simulink model "cartpole"  (R2021a)
settings: Solver=FixedStepAuto  StartTime=0.0  StopTime=T_end  FixedStep=Tsim  RelTol=1e-3
values from neighbouring files (symbols this model uses):
  r1 = const(1)    [loop_loader.m]
  r2 = const(2)    [loop_loader.m]
  Ts = 1e-2    (= 0.01)    [loop_loader.m]
undefined symbols (not defined in the file or in its folder): A, B, C, K_lqr, P_k_init, q1, q2, Q_ctrl, R_ctrl, x0
libraries: simulink x4
settings Model: Creator=rodpod21  LastModifiedBy=rodpod21

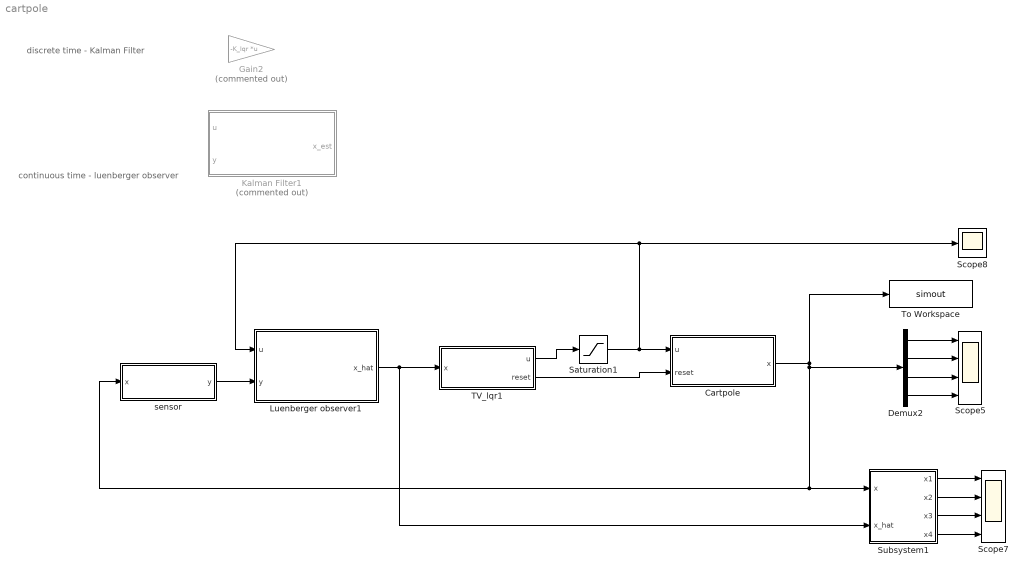
== system cartpole ==
  note: continuous time - luenberger observer
  note: discrete time - Kalman Filter
  Cartpole : Subsystem
  Demux2 : Demux
  Gain2 : Gain  Commented=on  Gain=-K_lqr  Multiplication=Matrix(K*u)
  Kalman Filter1 : Subsystem  Commented=on  TreatAsAtomicUnit=on  SystemSampleTime=Ts
  Luenberger observer1 : Subsystem
  Saturation1 : Saturate  UpperLimit=10  LowerLimit=-10
  Scope5 : Scope  NumInputPorts=4
  Scope7 : Scope  NumInputPorts=4
  Scope8 : Scope
  Subsystem1 : Subsystem
  TV_lqr1 : Subsystem  TreatAsAtomicUnit=on  SystemSampleTime=Ts
  To Workspace : ToWorkspace  VariableName=simout  SaveFormat=Timeseries  SampleTime=-1
  sensor : Subsystem
  wires:
  Subsystem1/1(x1) -> Scope7/1
  Subsystem1/3(x3) -> Scope7/3
  Subsystem1/4(x4) -> Scope7/4
  Subsystem1/2(x2) -> Scope7/2
  Demux2/4 -> Scope5/4
  Demux2/3 -> Scope5/3
  Demux2/2 -> Scope5/2
  Demux2/1 -> Scope5/1
  Saturation1/1 -> Cartpole/1(u), Scope8/1, Luenberger observer1/1(u)
  Luenberger observer1/1(x_hat) -> TV_lqr1/1(x), Subsystem1/2(x_hat)
  sensor/1(y) -> Luenberger observer1/2(y)
  TV_lqr1/1(u) -> Saturation1/1
  Cartpole/1(x) -> To Workspace/1, sensor/1(x), Subsystem1/1(x), Demux2/1
  TV_lqr1/2(reset) -> Cartpole/2(reset)

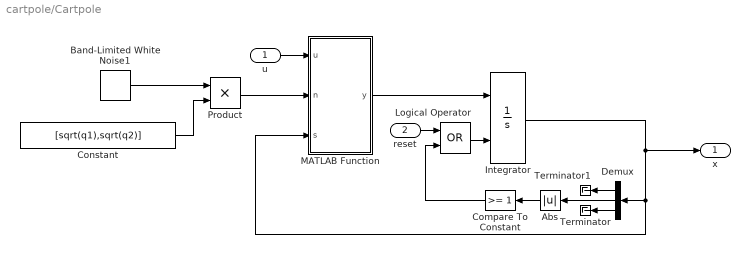
== system cartpole/Cartpole ==
  u : Inport
  reset : Inport  Port=2
  Abs : Abs
  Band-Limited White Noise1 : simulink/Sources/Band-Limited White Noise  Cov=[1,1]  Ts=Ts  seed=[23341]
  Compare To Constant : simulink/Logic and Bit Operations/Compare To Constant  relop=>=  const=1  OutDataTypeStr=boolean
  Constant : Constant  Value=[sqrt(q1),sqrt(q2)]
  Demux : Demux  Outputs=[2,1,1]
  Integrator : Integrator  ExternalReset=rising  InitialCondition=x0
  Logical Operator : Logic  Operator=OR  AllPortsSameDT=off  OutDataTypeStr=boolean
  MATLAB Function : MATLAB Function  TreatAsAtomicUnit=on
  Product : Product
  Terminator : Terminator
  Terminator1 : Terminator
  x : Outport
  wires:
  MATLAB Function/1(y) -> Integrator/1
  Integrator/1 -> x/1, MATLAB Function/3(s), Demux/1
  u/1 -> MATLAB Function/1(u)
  Band-Limited White Noise1/1 -> Product/1
  Product/1 -> MATLAB Function/2(n)
  Compare To Constant/1 -> Logical Operator/2
  Demux/3 -> Terminator/1
  Demux/1 -> Terminator1/1
  Demux/2 -> Abs/1
  Abs/1 -> Compare To Constant/1
  Logical Operator/1 -> Integrator/2
  reset/1 -> Logical Operator/1
  Constant/1 -> Product/2

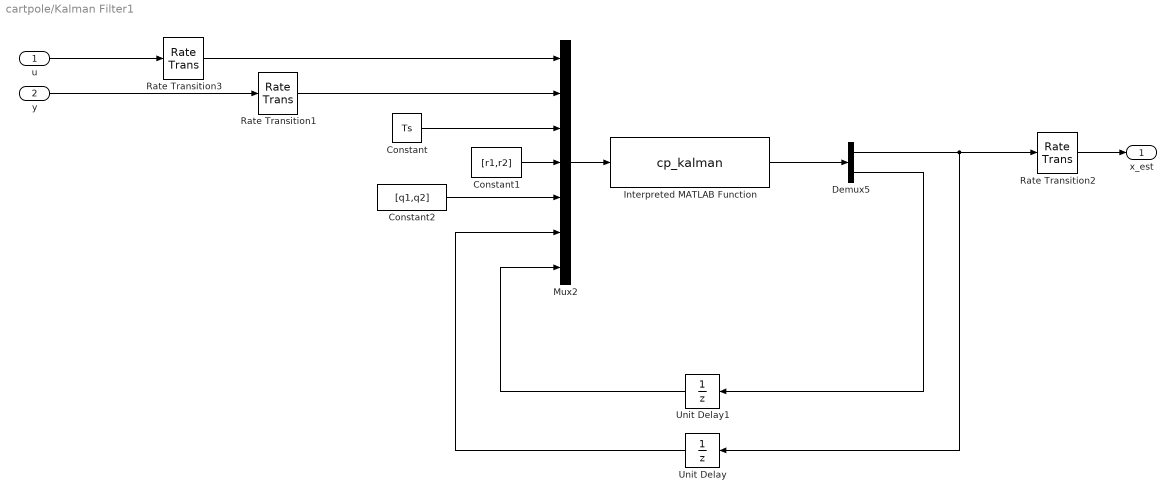
== system cartpole/Kalman Filter1 ==
  u : Inport
  y : Inport  Port=2
  Constant : Constant  Value=Ts
  Constant1 : Constant  Value=[r1,r2]
  Constant2 : Constant  Value=[q1,q2]
  Demux5 : Demux  Outputs=[4, 16]
  Interpreted MATLAB Function : MATLABFcn  MATLABFcn=cp_kalman  OutputDimensions=20
  Mux2 : Mux  Inputs=7
  Rate Transition1 : RateTransition  OutPortSampleTime=Ts
  Rate Transition2 : RateTransition
  Rate Transition3 : RateTransition  OutPortSampleTime=Ts
  Unit Delay : UnitDelay  InitialCondition=x0  SampleTime=-1  HasFrameUpgradeWarning=on
  Unit Delay1 : UnitDelay  InitialCondition=reshape( P_k_init*eye(4),[16,1])  SampleTime=-1  HasFrameUpgradeWarning=on
  x_est : Outport
  wires:
  Unit Delay1/1 -> Mux2/7
  Demux5/1 -> Rate Transition2/1, Unit Delay/1
  y/1 -> Rate Transition1/1
  Demux5/2 -> Unit Delay1/1
  Interpreted MATLAB Function/1 -> Demux5/1
  u/1 -> Rate Transition3/1
  Unit Delay/1 -> Mux2/6
  Mux2/1 -> Interpreted MATLAB Function/1
  Constant/1 -> Mux2/3
  Constant1/1 -> Mux2/4
  Constant2/1 -> Mux2/5
  Rate Transition3/1 -> Mux2/1
  Rate Transition1/1 -> Mux2/2
  Rate Transition2/1 -> x_est/1

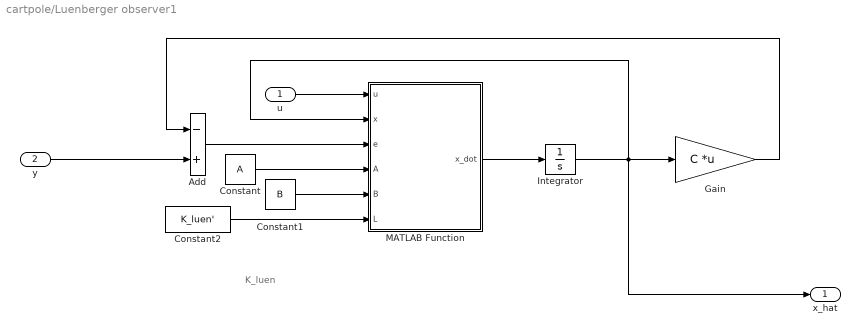
== system cartpole/Luenberger observer1 ==
  note: K_luen
  u : Inport
  y : Inport  Port=2
  Add : Sum  Inputs=-+
  Constant : Constant  Value=A
  Constant1 : Constant  Value=B
  Constant2 : Constant  Value=K_luen'
  Gain : Gain  Gain=C  Multiplication=Matrix(K*u)
  Integrator : Integrator  InitialCondition=[0,0,0,0]
  MATLAB Function : MATLAB Function  TreatAsAtomicUnit=on
  x_hat : Outport
  wires:
  y/1 -> Add/2
  u/1 -> MATLAB Function/1(u)
  Add/1 -> MATLAB Function/3(e)
  Gain/1 -> Add/1
  Integrator/1 -> x_hat/1, Gain/1, MATLAB Function/2(x)
  MATLAB Function/1(x_dot) -> Integrator/1
  Constant2/1 -> MATLAB Function/6(L)
  Constant1/1 -> MATLAB Function/5(B)
  Constant/1 -> MATLAB Function/4(A)

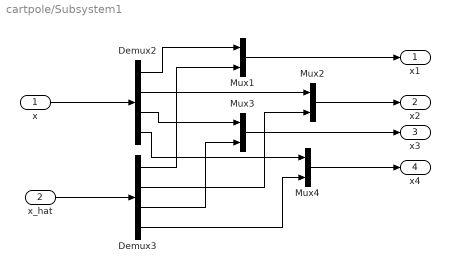
== system cartpole/Subsystem1 ==
  x : Inport
  x_hat : Inport  Port=2
  Demux2 : Demux
  Demux3 : Demux
  Mux{1..4} (4 alike) : Mux  Inputs=2
  x1 : Outport
  x2 : Outport  Port=2
  x3 : Outport  Port=3
  x4 : Outport  Port=4
  wires:
  Demux2/3 -> Mux3/1
  Demux3/4 -> Mux4/2
  x/1 -> Demux2/1
  Mux2/1 -> x2/1
  Demux2/1 -> Mux1/1
  x_hat/1 -> Demux3/1
  Demux3/2 -> Mux2/2
  Demux2/4 -> Mux4/1
  Demux3/3 -> Mux3/2
  Demux2/2 -> Mux2/1
  Mux3/1 -> x3/1
  Demux3/1 -> Mux1/2
  Mux4/1 -> x4/1
  Mux1/1 -> x1/1

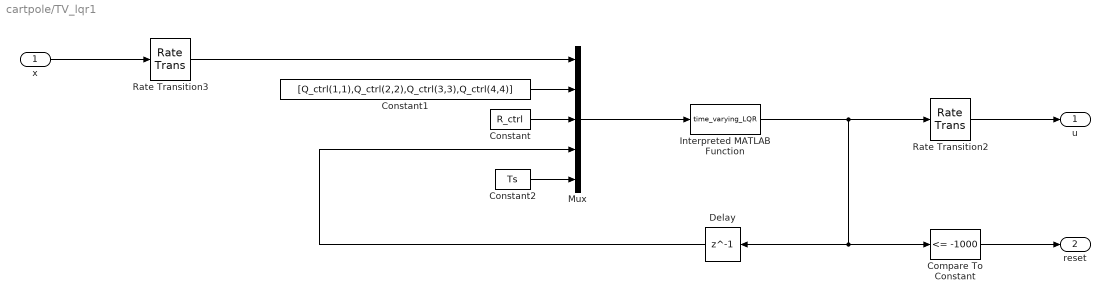
== system cartpole/TV_lqr1 ==
  x : Inport
  Compare To Constant : simulink/Logic and Bit Operations/Compare To Constant  relop=<=  const=-1000  OutDataTypeStr=boolean
  Constant : Constant  Value=R_ctrl
  Constant1 : Constant  Value=[Q_ctrl(1,1),Q_ctrl(2,2),Q_ctrl(3,3),Q_ctrl(4,4)]
  Constant2 : Constant  Value=Ts
  Delay : Delay  DelayLength=1  InitialCondition=0
  Interpreted MATLAB Function : MATLABFcn  MATLABFcn=time_varying_LQR
  Mux : Mux  Inputs=5
  Rate Transition2 : RateTransition
  Rate Transition3 : RateTransition  OutPortSampleTime=Ts
  u : Outport
  reset : Outport  Port=2
  wires:
  Constant2/1 -> Mux/5
  Rate Transition2/1 -> u/1
  Rate Transition3/1 -> Mux/1
  Delay/1 -> Mux/4
  Constant1/1 -> Mux/2
  Constant/1 -> Mux/3
  Mux/1 -> Interpreted MATLAB Function/1
  x/1 -> Rate Transition3/1
  Interpreted MATLAB Function/1 -> Rate Transition2/1, Compare To Constant/1, Delay/1
  Compare To Constant/1 -> reset/1

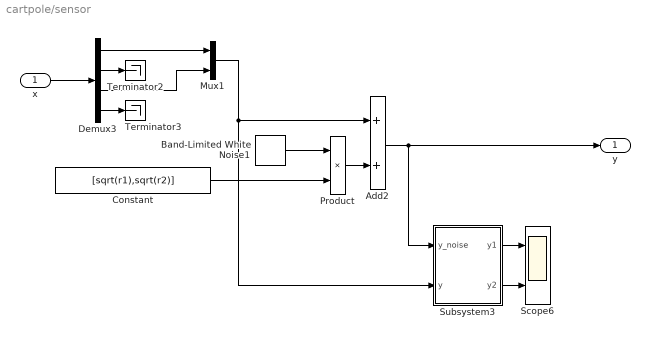
== system cartpole/sensor ==
  x : Inport
  Add2 : Sum
  Band-Limited White Noise1 : simulink/Sources/Band-Limited White Noise  Cov=[1,1]  Ts=Ts  seed=[8451]
  Constant : Constant  Value=[sqrt(r1),sqrt(r2)]
  Demux3 : Demux
  Mux1 : Mux  Inputs=2
  Product : Product
  Scope6 : Scope  NumInputPorts=2
  Subsystem3 : Subsystem
  Terminator2 : Terminator
  Terminator3 : Terminator
  y : Outport
  wires:
  Demux3/4 -> Terminator3/1
  Demux3/2 -> Terminator2/1
  Demux3/3 -> Mux1/2
  Add2/1 -> y/1, Subsystem3/1(y_noise)
  Subsystem3/2(y2) -> Scope6/2
  x/1 -> Demux3/1
  Mux1/1 -> Subsystem3/2(y), Add2/1
  Subsystem3/1(y1) -> Scope6/1
  Demux3/1 -> Mux1/1
  Product/1 -> Add2/2
  Band-Limited White Noise1/1 -> Product/1
  Constant/1 -> Product/2

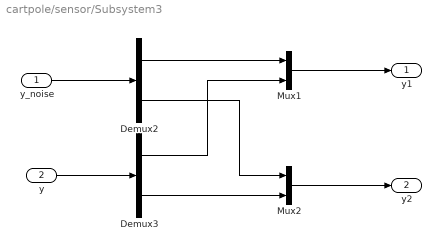
== system cartpole/sensor/Subsystem3 ==
  y_noise : Inport
  y : Inport  Port=2
  Demux2 : Demux  Outputs=2
  Demux3 : Demux  Outputs=2
  Mux1 : Mux  Inputs=2
  Mux2 : Mux  Inputs=2
  y1 : Outport
  y2 : Outport  Port=2
  wires:
  Mux1/1 -> y1/1
  Demux3/1 -> Mux1/2
  Demux2/2 -> Mux2/1
  Demux3/2 -> Mux2/2
  y/1 -> Demux3/1
  Demux2/1 -> Mux1/1
  Mux2/1 -> y2/1
  y_noise/1 -> Demux2/1

== matlab function cartpole/Luenberger observer1/MATLAB Function ==
  data: u input; x_dot output; x input; e input; A input; B input; L input
function x_dot = fcn(u,x,e,A,B,L)

x_dot = A*x + B*u + L*e;

== matlab function cartpole/Cartpole/MATLAB Function ==
  data: u input; n input; s input; y output
function y = fcn(u,n,s)

dot_x = s(2) ;
theta = s(3) ;
dot_theta = s(4) ;

m = 0.1;
L = 1;
g = 9.81;
M = 1;
d1 = 1;
d2 = 0.5;


x_ddot = u  + m*L*dot_theta^2 * sin(theta) - m*g*cos(theta) *  sin(theta) ;
x_ddot = x_ddot / ( M+m-m* cos(theta)^2 )  + n(1) - d1*dot_x;

theta_ddot = (g*sin( theta ) -  cos( theta )*x_ddot ) / L  + n(2) - d2*dot_theta ;


y = [ dot_x, x_ddot , dot_theta, theta_ddot  ];
